simulink model "atrias_system_testing_delay"  (R2014a)
settings: Solver=FixedStepDiscrete  StartTime=0.0  StopTime=inf  FixedStep=sample_time  RelTol=1e-3
PreLoadFcn:
  | set_sampletime
PostLoadFcn:
  | set_sampletime
InitFcn:
  | sys_params
StartFcn:
  | set_sampletime
values from neighbouring files (symbols this model uses):
  A_lpf_velocity = 1 + B1_lpf_velocity + B2_lpf_velocity    [daq_params_osu.m]
  B1_lpf_velocity = -2*exp(-lpf_damping*fcut_velocity*sample_time)*cos(fcut_velocity*sample_time*sqrt(1-lpf_damping^2))    [daq_params_osu.m]
  B2_lpf_velocity = exp(-2*lpf_damping*fcut_velocity*sample_time)    [daq_params_osu.m]
  BOOM_MAX_ENCODER_TICKS = 2^17 - 1    (= 131071)    [daq_params_osu.m]
  BOOM_PITCH_CAL_VALUE_RAD = 0    [daq_params_osu.m]
  BOOM_PITCH_CAL_VALUE_TICKS = 43809    [daq_params_osu.m]
  BOOM_PITCH_ENCODER_RAD_PER_TICK = -2*pi / (2^17 * 2)    (= -2.39684498107e-05)    [daq_params_osu.m]
  BOOM_ROLL_CAL_VALUE_RAD = 0.1271    [daq_params_osu.m]
  BOOM_ROLL_CAL_VALUE_TICKS = 9318    [daq_params_osu.m]
  BOOM_ROLL_ENCODER_RAD_PER_TICK = 2*pi / (2^17 * 7)    (= 6.84812851735e-06)    [daq_params_osu.m]
  BOOM_YAW_ENCODER_RAD_PER_TICK = 2*pi / (2^17 * 9.6)    (= 4.9934270439e-06)    [daq_params_osu.m]
  CURRENT_LIMIT = 100    [daq_params_osu.m]
  fcut_smooth = 16*(2*pi)    (= 100.530964915)    [daq_params_osu.m]
  fcut_unwrap = 8*(2*pi)    (= 50.2654824574)    [daq_params_osu.m]
  gui_disable_cmd = 0    [daq_params_osu.m]
  gui_enable_cmd = 0    [daq_params_osu.m]
  gui_estop_cmd = 0    [daq_params_osu.m]
  gui_reset_cmd = 0    [daq_params_osu.m]
  HIP_ABS_ENCODER_RAD_PER_TICK = 2*pi / 2^13    (= 0.000766990393943)    [daq_params_osu.m]
  HIP_ABS_MAX_ENCODER_TICKS = 2^13 - 1    (= 8191)    [daq_params_osu.m]
  HIP_INC_ENCODER_RAD_PER_TICK = 2*pi / (2500 * 4 * 57)    (= 1.10231321179e-05)    [daq_params_osu.m]
  HIP_INC_MAX_ENCODER_TICKS = 2^16 - 1    (= 65535)    [daq_params_osu.m]
  HIP_MOTOR_CONSTANT = 0.184    [daq_params_osu.m]
  HIP_MTR_GEAR_RATIO = 57    [daq_params_osu.m]
  HIP_MTR_MAX_TORQUE = MTR_HIP_MAX_CURRENT*HIP_MOTOR_CONSTANT*HIP_MTR_GEAR_RATIO    (= 629.28)    [daq_params_osu.m]
  INC_ENC_DIRS = -[ LEG1_MOTOR_A_DIRECTION ... (first row only)    [daq_params_osu.m]
  INC_ENC_RAD_PER_TICK = 2*pi/14000/LEG_MTR_GEAR_RATIO    (= 8.97597901026e-06)    [daq_params_osu.m]
  k_sea = 4118    [sys_params.m]
  LEFT_HIP_CALIB_POS = 0    [daq_params_osu.m]
  LEFT_HIP_CALIB_VAL = 7192 - 2^13    (= -1000)    [daq_params_osu.m]
  LEFT_MOTOR_HIP_DIRECTION = -1.0    (= -1)    [daq_params_osu.m]
  LEG1_LEG_A_CALIB_VAL = 265417675    [daq_params_osu.m]
  LEG1_LEG_A_RAD_PER_CNT = -9.8039216e-09    [daq_params_osu.m]
  LEG1_LEG_B_CALIB_VAL = 175319150    [daq_params_osu.m]
  LEG1_LEG_B_RAD_PER_CNT = -9.8039216e-09    [daq_params_osu.m]
  LEG1_MOTOR_A_DIRECTION = -1.0    (= -1)    [daq_params_osu.m]
  LEG1_MOTOR_B_DIRECTION = -1.0    (= -1)    [daq_params_osu.m]
  LEG1_TRAN_A_CALIB_VAL = 143046540    [daq_params_osu.m]
  LEG1_TRAN_A_RAD_PER_CNT = 9.8039216e-09    [daq_params_osu.m]
  LEG1_TRAN_B_CALIB_VAL = 142356572    [daq_params_osu.m]
  LEG1_TRAN_B_RAD_PER_CNT = -9.8039216e-09    [daq_params_osu.m]
  LEG2_LEG_A_CALIB_VAL = 264357825    [daq_params_osu.m]
  LEG2_LEG_A_RAD_PER_CNT = -9.8039216e-09    [daq_params_osu.m]
  LEG2_LEG_B_CALIB_VAL = 261444054    [daq_params_osu.m]
  LEG2_LEG_B_RAD_PER_CNT = 9.8039216e-09    [daq_params_osu.m]
  LEG2_MOTOR_A_DIRECTION = 1.0    (= 1)    [daq_params_osu.m]
  LEG2_MOTOR_B_DIRECTION = 1.0    (= 1)    [daq_params_osu.m]
  LEG2_TRAN_A_CALIB_VAL = 142300933    [daq_params_osu.m]
  LEG2_TRAN_A_RAD_PER_CNT = 9.8039216e-09    [daq_params_osu.m]
  LEG2_TRAN_B_CALIB_VAL = 142287413    [daq_params_osu.m]
  LEG2_TRAN_B_RAD_PER_CNT = -9.8039216e-09    [daq_params_osu.m]
  LEG_A_CALIB_LOC = pi + 0.305432619099008    (= 3.44702527269)    [daq_params_osu.m]
  LEG_B_CALIB_LOC = pi - 0.305432619099008    (= 2.83616003449)    [daq_params_osu.m]
  LEG_MOTOR_CONSTANT = 0.119    [daq_params_osu.m]
  LEG_MTR_GEAR_RATIO = 50    [daq_params_osu.m]
  LEG_MTR_MAX_TORQUE = MTR_MAX_CURRENT*LEG_MOTOR_CONSTANT*LEG_MTR_GEAR_RATIO    (= 922.25)    [daq_params_osu.m]
  max_encoder_velocity = 200    [daq_params_osu.m]
  MEDULLA_ADC_MAX_VOLTS = 2.70    (= 2.7)    [daq_params_osu.m]
  MEDULLA_ADC_OFFSET_COUNTS = 172    [daq_params_osu.m]
  MEDULLA_STATE_ERROR = 5    [daq_params_osu.m]
  MEDULLA_STATE_HALT = 4    [daq_params_osu.m]
  MEDULLA_STATE_IDLE = 0    [daq_params_osu.m]
  MEDULLA_STATE_RESET = 6    [daq_params_osu.m]
  MEDULLA_STATE_RUN = 2    [daq_params_osu.m]
  MEDULLA_TIMER_FREQ = 32e6    (= 32000000)    [daq_params_osu.m]
  MOTOR_POSITION_LIMITS_LOWER = [2.5; 1.4; 0.4]    [daq_params_osu.m]
  MOTOR_POSITION_LIMITS_UPPER = [4.9; 3.8; 2.5]    [daq_params_osu.m]
  MTR_HIP_MAX_CURRENT = 60.0    (= 60)    [daq_params_osu.m]
  MTR_MAX_CONT_CURRENT = 100.0    (= 100)    [daq_params_osu.m]
  MTR_MAX_COUNT = 19900    [daq_params_osu.m]
  MTR_MAX_CURRENT = 155.0    (= 155)    [daq_params_osu.m]
  nom_sample_time = 0.001    [sys_params.m]
  RIGHT_HIP_CALIB_POS = 0    [daq_params_osu.m]
  RIGHT_HIP_CALIB_VAL = 1091    [daq_params_osu.m]
  RIGHT_MOTOR_HIP_DIRECTION = 1.0    (= 1)    [daq_params_osu.m]
  sample_time = 1/update_freq    (= 0.001)    [daq_params_osu.m]
  sensor_start_time = 8    [daq_params_osu.m]
undefined symbols (not defined in the file or in its folder): max_sensor_velocity
libraries: xpcethercatlib x196, simulink x50, slrtlib x4, dspswit3 x1
(part 3 of 4)

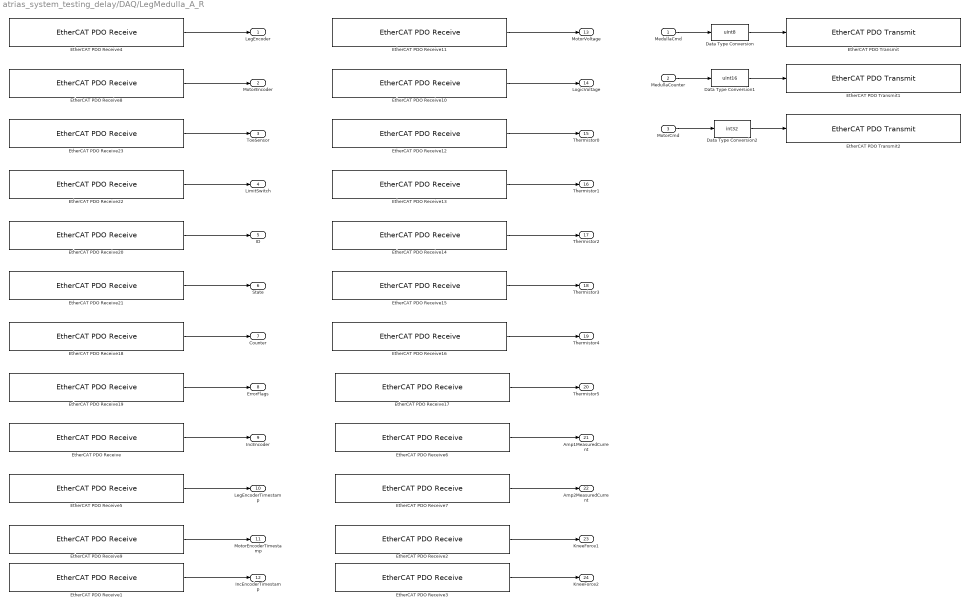
== system atrias_system_testing_delay/DAQ/LegMedulla_A_R ==
  MedullaCmd : Inport
  MedullaCounter : Inport  Port=2
  MotorCmd : Inport  Port=3
  Data Type Conversion : DataTypeConversion  OutDataTypeStr=uint8
  Data Type Conversion1 : DataTypeConversion  OutDataTypeStr=uint16
  Data Type Conversion2 : DataTypeConversion  OutDataTypeStr=int32
  EtherCAT PDO Receive : xpcethercatlib/EtherCAT PDO Receive  Priority=2  sig_name=Box 7 (ATRIAS 2.1 Leg (Medulla 1.5)).Incremental Encoder.Incremental Encoder  sig_offset=2120  sig_type=uint16  type_size=16  sig_dim=1  device_id=0  sample_time=0.001000
  EtherCAT PDO Receive1 : xpcethercatlib/EtherCAT PDO Receive  Priority=2  sig_name=Box 7 (ATRIAS 2.1 Leg (Medulla 1.5)).Incremental Encoder.Incremental Encoder Timestamp  sig_offset=2136  sig_type=uint16  type_size=16  sig_dim=1  device_id=0  sample_time=0.001000
  EtherCAT PDO Receive10 : xpcethercatlib/EtherCAT PDO Receive  Priority=2  sig_name=Box 7 (ATRIAS 2.1 Leg (Medulla 1.5)).Power.Logic Voltage  sig_offset=2168  sig_type=uint16  type_size=16  sig_dim=1  device_id=0  sample_time=0.001000
  EtherCAT PDO Receive11 : xpcethercatlib/EtherCAT PDO Receive  Priority=2  sig_name=Box 7 (ATRIAS 2.1 Leg (Medulla 1.5)).Power.Motor Voltage  sig_offset=2152  sig_type=uint16  type_size=16  sig_dim=1  device_id=0  sample_time=0.001000
  EtherCAT PDO Receive12 : xpcethercatlib/EtherCAT PDO Receive  Priority=2  sig_name=Box 7 (ATRIAS 2.1 Leg (Medulla 1.5)).Thermistors.Thermistor 0  sig_offset=2184  sig_type=uint16  type_size=16  sig_dim=1  device_id=0  sample_time=0.001000
  EtherCAT PDO Receive13 : xpcethercatlib/EtherCAT PDO Receive  Priority=2  sig_name=Box 7 (ATRIAS 2.1 Leg (Medulla 1.5)).Thermistors.Thermistor 1  sig_offset=2200  sig_type=uint16  type_size=16  sig_dim=1  device_id=0  sample_time=0.001000
  EtherCAT PDO Receive14 : xpcethercatlib/EtherCAT PDO Receive  Priority=2  sig_name=Box 7 (ATRIAS 2.1 Leg (Medulla 1.5)).Thermistors.Thermistor 2  sig_offset=2216  sig_type=uint16  type_size=16  sig_dim=1  device_id=0  sample_time=0.001000
  EtherCAT PDO Receive15 : xpcethercatlib/EtherCAT PDO Receive  Priority=2  sig_name=Box 7 (ATRIAS 2.1 Leg (Medulla 1.5)).Thermistors.Thermistor 3  sig_offset=2232  sig_type=uint16  type_size=16  sig_dim=1  device_id=0  sample_time=0.001000
  EtherCAT PDO Receive16 : xpcethercatlib/EtherCAT PDO Receive  Priority=2  sig_name=Box 7 (ATRIAS 2.1 Leg (Medulla 1.5)).Thermistors.Thermistor 4  sig_offset=2248  sig_type=uint16  type_size=16  sig_dim=1  device_id=0  sample_time=0.001000
  EtherCAT PDO Receive17 : xpcethercatlib/EtherCAT PDO Receive  Priority=2  sig_name=Box 7 (ATRIAS 2.1 Leg (Medulla 1.5)).Thermistors.Thermistor 5  sig_offset=2264  sig_type=uint16  type_size=16  sig_dim=1  device_id=0  sample_time=0.001000
  EtherCAT PDO Receive18 : xpcethercatlib/EtherCAT PDO Receive  Priority=2  sig_name=Box 7 (ATRIAS 2.1 Leg (Medulla 1.5)).uController Status.Counter  sig_offset=1984  sig_type=uint8  type_size=8  sig_dim=1  device_id=0  sample_time=0.001000
  EtherCAT PDO Receive19 : xpcethercatlib/EtherCAT PDO Receive  Priority=2  sig_name=Box 7 (ATRIAS 2.1 Leg (Medulla 1.5)).uController Status.Error Flags  sig_offset=1992  sig_type=uint8  type_size=8  sig_dim=1  device_id=0  sample_time=0.001000
  EtherCAT PDO Receive2 : xpcethercatlib/EtherCAT PDO Receive  Priority=2  sig_name=Box 7 (ATRIAS 2.1 Leg (Medulla 1.5)).Knee Force.Knee Force 1  sig_offset=2312  sig_type=uint16  type_size=16  sig_dim=1  device_id=0  sample_time=0.001000
  EtherCAT PDO Receive20 : xpcethercatlib/EtherCAT PDO Receive  Priority=2  sig_name=Box 7 (ATRIAS 2.1 Leg (Medulla 1.5)).uController Status.ID  sig_offset=1968  sig_type=uint8  type_size=8  sig_dim=1  device_id=0  sample_time=0.001000
  EtherCAT PDO Receive21 : xpcethercatlib/EtherCAT PDO Receive  Priority=2  sig_name=Box 7 (ATRIAS 2.1 Leg (Medulla 1.5)).uController Status.State  sig_offset=1976  sig_type=uint8  type_size=8  sig_dim=1  device_id=0  sample_time=0.001000
  EtherCAT PDO Receive22 : xpcethercatlib/EtherCAT PDO Receive  Priority=2  sig_name=Box 7 (ATRIAS 2.1 Leg (Medulla 1.5)).uController Status.Limit Switch  sig_offset=2000  sig_type=uint8  type_size=8  sig_dim=1  device_id=0  sample_time=0.001000
  EtherCAT PDO Receive23 : xpcethercatlib/EtherCAT PDO Receive  Priority=2  sig_name=Box 7 (ATRIAS 2.1 Leg (Medulla 1.5)).uController Status.Toe Sensor  sig_offset=2008  sig_type=uint16  type_size=16  sig_dim=1  device_id=0  sample_time=0.001000
  EtherCAT PDO Receive3 : xpcethercatlib/EtherCAT PDO Receive  Priority=2  sig_name=Box 7 (ATRIAS 2.1 Leg (Medulla 1.5)).Knee Force.Knee Force 2  sig_offset=2328  sig_type=uint16  type_size=16  sig_dim=1  device_id=0  sample_time=0.001000
  EtherCAT PDO Receive4 : xpcethercatlib/EtherCAT PDO Receive  Priority=2  sig_name=Box 7 (ATRIAS 2.1 Leg (Medulla 1.5)).Leg Encoder.Leg Encoder  sig_offset=2072  sig_type=uint32  type_size=32  sig_dim=1  device_id=0  sample_time=0.001000
  EtherCAT PDO Receive5 : xpcethercatlib/EtherCAT PDO Receive  Priority=2  sig_name=Box 7 (ATRIAS 2.1 Leg (Medulla 1.5)).Leg Encoder.Leg Encoder Timestamp  sig_offset=2104  sig_type=uint16  type_size=16  sig_dim=1  device_id=0  sample_time=0.001000
  EtherCAT PDO Receive6 : xpcethercatlib/EtherCAT PDO Receive  Priority=2  sig_name=Box 7 (ATRIAS 2.1 Leg (Medulla 1.5)).Measured Current.Amp 1 Measured Current  sig_offset=2280  sig_type=int16  type_size=16  sig_dim=1  device_id=0  sample_time=0.001000
  EtherCAT PDO Receive7 : xpcethercatlib/EtherCAT PDO Receive  Priority=2  sig_name=Box 7 (ATRIAS 2.1 Leg (Medulla 1.5)).Measured Current.Amp 2 Measured Current  sig_offset=2296  sig_type=int16  type_size=16  sig_dim=1  device_id=0  sample_time=0.001000
  EtherCAT PDO Receive8 : xpcethercatlib/EtherCAT PDO Receive  Priority=2  sig_name=Box 7 (ATRIAS 2.1 Leg (Medulla 1.5)).Motor Encoder.Motor Encoder  sig_offset=2024  sig_type=uint32  type_size=32  sig_dim=1  device_id=0  sample_time=0.001000
  EtherCAT PDO Receive9 : xpcethercatlib/EtherCAT PDO Receive  Priority=2  sig_name=Box 7 (ATRIAS 2.1 Leg (Medulla 1.5)).Motor Encoder.Motor Encoder Timestamp  sig_offset=2056  sig_type=uint16  type_size=16  sig_dim=1  device_id=0  sample_time=0.001000
  EtherCAT PDO Transmit : xpcethercatlib/EtherCAT PDO Transmit   Priority=3  sig_name=Box 7 (ATRIAS 2.1 Leg (Medulla 1.5)).uControllerInput.Command  sig_offset=1968  sig_type=uint8  type_size=8  sig_dim=1  device_id=0  sample_time=0.001000
  EtherCAT PDO Transmit1 : xpcethercatlib/EtherCAT PDO Transmit   Priority=3  sig_name=Box 7 (ATRIAS 2.1 Leg (Medulla 1.5)).uControllerInput.Counter  sig_offset=1976  sig_type=uint16  type_size=16  sig_dim=1  device_id=0  sample_time=0.001000
  EtherCAT PDO Transmit2 : xpcethercatlib/EtherCAT PDO Transmit   Priority=3  sig_name=Box 7 (ATRIAS 2.1 Leg (Medulla 1.5)).uControllerInput.Motor Current  sig_offset=1992  sig_type=int32  type_size=32  sig_dim=1  device_id=0  sample_time=0.001000
  LegEncoder : Outport
  MotorEncoder : Outport  Port=2
  ToeSensor : Outport  Port=3
  LimitSwitch : Outport  Port=4
  ID : Outport  Port=5
  State : Outport  Port=6
  Counter : Outport  Port=7
  ErrorFlags : Outport  Port=8
  IncEncoder : Outport  Port=9
  LegEncoderTimestamp : Outport  Port=10
  MotorEncoderTimestamp : Outport  Port=11
  IncEncoderTimestamp : Outport  Port=12
  MotorVoltage : Outport  Port=13
  LogicVoltage : Outport  Port=14
  Thermistor0 : Outport  Port=15
  Thermistor1 : Outport  Port=16
  Thermistor2 : Outport  Port=17
  Thermistor3 : Outport  Port=18
  Thermistor4 : Outport  Port=19
  Thermistor5 : Outport  Port=20
  Amp1MeasuredCurrent : Outport  Port=21
  Amp2MeasuredCurrent : Outport  Port=22
  KneeForce1 : Outport  Port=23
  KneeForce2 : Outport  Port=24
  wires:
  Data Type Conversion/1 -> EtherCAT PDO Transmit/1
  Data Type Conversion1/1 -> EtherCAT PDO Transmit1/1
  Data Type Conversion2/1 -> EtherCAT PDO Transmit2/1
  EtherCAT PDO Receive/1 -> IncEncoder/1
  EtherCAT PDO Receive1/1 -> IncEncoderTimestamp/1
  EtherCAT PDO Receive2/1 -> KneeForce1/1
  EtherCAT PDO Receive3/1 -> KneeForce2/1
  EtherCAT PDO Receive4/1 -> LegEncoder/1
  EtherCAT PDO Receive5/1 -> LegEncoderTimestamp/1
  EtherCAT PDO Receive6/1 -> Amp1MeasuredCurrent/1
  EtherCAT PDO Receive7/1 -> Amp2MeasuredCurrent/1
  EtherCAT PDO Receive8/1 -> MotorEncoder/1
  EtherCAT PDO Receive9/1 -> MotorEncoderTimestamp/1
  EtherCAT PDO Receive10/1 -> LogicVoltage/1
  EtherCAT PDO Receive11/1 -> MotorVoltage/1
  EtherCAT PDO Receive12/1 -> Thermistor0/1
  EtherCAT PDO Receive13/1 -> Thermistor1/1
  EtherCAT PDO Receive14/1 -> Thermistor2/1
  EtherCAT PDO Receive15/1 -> Thermistor3/1
  EtherCAT PDO Receive16/1 -> Thermistor4/1
  EtherCAT PDO Receive17/1 -> Thermistor5/1
  EtherCAT PDO Receive18/1 -> Counter/1
  EtherCAT PDO Receive19/1 -> ErrorFlags/1
  EtherCAT PDO Receive20/1 -> ID/1
  EtherCAT PDO Receive22/1 -> LimitSwitch/1
  EtherCAT PDO Receive21/1 -> State/1
  EtherCAT PDO Receive23/1 -> ToeSensor/1
  MedullaCmd/1 -> Data Type Conversion/1
  MedullaCounter/1 -> Data Type Conversion1/1
  MotorCmd/1 -> Data Type Conversion2/1

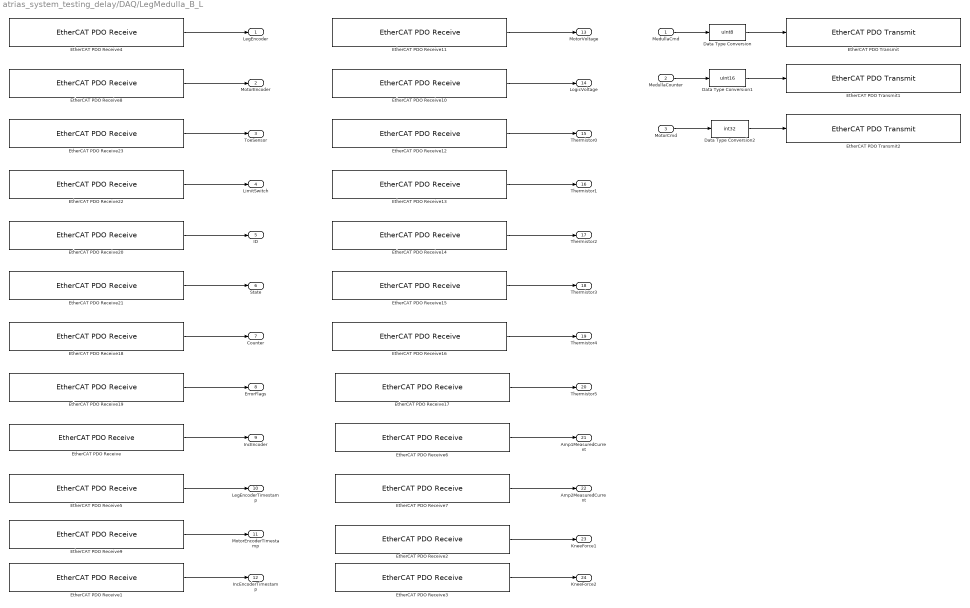
== system atrias_system_testing_delay/DAQ/LegMedulla_B_L ==
  MedullaCmd : Inport
  MedullaCounter : Inport  Port=2
  MotorCmd : Inport  Port=3
  Data Type Conversion : DataTypeConversion  OutDataTypeStr=uint8
  Data Type Conversion1 : DataTypeConversion  OutDataTypeStr=uint16
  Data Type Conversion2 : DataTypeConversion  OutDataTypeStr=int32
  EtherCAT PDO Receive : xpcethercatlib/EtherCAT PDO Receive  Priority=2  sig_name=Box 5 (ATRIAS 2.1 Leg (Medulla 1.5)).Incremental Encoder.Incremental Encoder  sig_offset=1368  sig_type=uint16  type_size=16  sig_dim=1  device_id=0  sample_time=0.001000
  EtherCAT PDO Receive1 : xpcethercatlib/EtherCAT PDO Receive  Priority=2  sig_name=Box 5 (ATRIAS 2.1 Leg (Medulla 1.5)).Incremental Encoder.Incremental Encoder Timestamp  sig_offset=1384  sig_type=uint16  type_size=16  sig_dim=1  device_id=0  sample_time=0.001000
  EtherCAT PDO Receive10 : xpcethercatlib/EtherCAT PDO Receive  Priority=2  sig_name=Box 5 (ATRIAS 2.1 Leg (Medulla 1.5)).Power.Logic Voltage  sig_offset=1416  sig_type=uint16  type_size=16  sig_dim=1  device_id=0  sample_time=0.001000
  EtherCAT PDO Receive11 : xpcethercatlib/EtherCAT PDO Receive  Priority=2  sig_name=Box 5 (ATRIAS 2.1 Leg (Medulla 1.5)).Power.Motor Voltage  sig_offset=1400  sig_type=uint16  type_size=16  sig_dim=1  device_id=0  sample_time=0.001000
  EtherCAT PDO Receive12 : xpcethercatlib/EtherCAT PDO Receive  Priority=2  sig_name=Box 5 (ATRIAS 2.1 Leg (Medulla 1.5)).Thermistors.Thermistor 0  sig_offset=1432  sig_type=uint16  type_size=16  sig_dim=1  device_id=0  sample_time=0.001000
  EtherCAT PDO Receive13 : xpcethercatlib/EtherCAT PDO Receive  Priority=2  sig_name=Box 5 (ATRIAS 2.1 Leg (Medulla 1.5)).Thermistors.Thermistor 1  sig_offset=1448  sig_type=uint16  type_size=16  sig_dim=1  device_id=0  sample_time=0.001000
  EtherCAT PDO Receive14 : xpcethercatlib/EtherCAT PDO Receive  Priority=2  sig_name=Box 5 (ATRIAS 2.1 Leg (Medulla 1.5)).Thermistors.Thermistor 2  sig_offset=1464  sig_type=uint16  type_size=16  sig_dim=1  device_id=0  sample_time=0.001000
  EtherCAT PDO Receive15 : xpcethercatlib/EtherCAT PDO Receive  Priority=2  sig_name=Box 5 (ATRIAS 2.1 Leg (Medulla 1.5)).Thermistors.Thermistor 3  sig_offset=1480  sig_type=uint16  type_size=16  sig_dim=1  device_id=0  sample_time=0.001000
  EtherCAT PDO Receive16 : xpcethercatlib/EtherCAT PDO Receive  Priority=2  sig_name=Box 5 (ATRIAS 2.1 Leg (Medulla 1.5)).Thermistors.Thermistor 4  sig_offset=1496  sig_type=uint16  type_size=16  sig_dim=1  device_id=0  sample_time=0.001000
  EtherCAT PDO Receive17 : xpcethercatlib/EtherCAT PDO Receive  Priority=2  sig_name=Box 5 (ATRIAS 2.1 Leg (Medulla 1.5)).Thermistors.Thermistor 5  sig_offset=1512  sig_type=uint16  type_size=16  sig_dim=1  device_id=0  sample_time=0.001000
  EtherCAT PDO Receive18 : xpcethercatlib/EtherCAT PDO Receive  Priority=2  sig_name=Box 5 (ATRIAS 2.1 Leg (Medulla 1.5)).uController Status.Counter  sig_offset=1232  sig_type=uint8  type_size=8  sig_dim=1  device_id=0  sample_time=0.001000
  EtherCAT PDO Receive19 : xpcethercatlib/EtherCAT PDO Receive  Priority=2  sig_name=Box 5 (ATRIAS 2.1 Leg (Medulla 1.5)).uController Status.Error Flags  sig_offset=1240  sig_type=uint8  type_size=8  sig_dim=1  device_id=0  sample_time=0.001000
  EtherCAT PDO Receive2 : xpcethercatlib/EtherCAT PDO Receive  Priority=2  sig_name=Box 5 (ATRIAS 2.1 Leg (Medulla 1.5)).Knee Force.Knee Force 1  sig_offset=1560  sig_type=uint16  type_size=16  sig_dim=1  device_id=0  sample_time=0.001000
  EtherCAT PDO Receive20 : xpcethercatlib/EtherCAT PDO Receive  Priority=2  sig_name=Box 5 (ATRIAS 2.1 Leg (Medulla 1.5)).uController Status.ID  sig_offset=1216  sig_type=uint8  type_size=8  sig_dim=1  device_id=0  sample_time=0.001000
  EtherCAT PDO Receive21 : xpcethercatlib/EtherCAT PDO Receive  Priority=2  sig_name=Box 5 (ATRIAS 2.1 Leg (Medulla 1.5)).uController Status.State  sig_offset=1224  sig_type=uint8  type_size=8  sig_dim=1  device_id=0  sample_time=0.001000
  EtherCAT PDO Receive22 : xpcethercatlib/EtherCAT PDO Receive  Priority=2  sig_name=Box 5 (ATRIAS 2.1 Leg (Medulla 1.5)).uController Status.Limit Switch  sig_offset=1248  sig_type=uint8  type_size=8  sig_dim=1  device_id=0  sample_time=0.001000
  EtherCAT PDO Receive23 : xpcethercatlib/EtherCAT PDO Receive  Priority=2  sig_name=Box 5 (ATRIAS 2.1 Leg (Medulla 1.5)).uController Status.Toe Sensor  sig_offset=1256  sig_type=uint16  type_size=16  sig_dim=1  device_id=0  sample_time=0.001000
  EtherCAT PDO Receive3 : xpcethercatlib/EtherCAT PDO Receive  Priority=2  sig_name=Box 5 (ATRIAS 2.1 Leg (Medulla 1.5)).Knee Force.Knee Force 2  sig_offset=1576  sig_type=uint16  type_size=16  sig_dim=1  device_id=0  sample_time=0.001000
  EtherCAT PDO Receive4 : xpcethercatlib/EtherCAT PDO Receive  Priority=2  sig_name=Box 5 (ATRIAS 2.1 Leg (Medulla 1.5)).Leg Encoder.Leg Encoder  sig_offset=1320  sig_type=uint32  type_size=32  sig_dim=1  device_id=0  sample_time=0.001000
  EtherCAT PDO Receive5 : xpcethercatlib/EtherCAT PDO Receive  Priority=2  sig_name=Box 5 (ATRIAS 2.1 Leg (Medulla 1.5)).Leg Encoder.Leg Encoder Timestamp  sig_offset=1352  sig_type=uint16  type_size=16  sig_dim=1  device_id=0  sample_time=0.001000
  EtherCAT PDO Receive6 : xpcethercatlib/EtherCAT PDO Receive  Priority=2  sig_name=Box 5 (ATRIAS 2.1 Leg (Medulla 1.5)).Measured Current.Amp 1 Measured Current  sig_offset=1528  sig_type=int16  type_size=16  sig_dim=1  device_id=0  sample_time=0.001000
  EtherCAT PDO Receive7 : xpcethercatlib/EtherCAT PDO Receive  Priority=2  sig_name=Box 5 (ATRIAS 2.1 Leg (Medulla 1.5)).Measured Current.Amp 2 Measured Current  sig_offset=1544  sig_type=int16  type_size=16  sig_dim=1  device_id=0  sample_time=0.001000
  EtherCAT PDO Receive8 : xpcethercatlib/EtherCAT PDO Receive  Priority=2  sig_name=Box 5 (ATRIAS 2.1 Leg (Medulla 1.5)).Motor Encoder.Motor Encoder  sig_offset=1272  sig_type=uint32  type_size=32  sig_dim=1  device_id=0  sample_time=0.001000
  EtherCAT PDO Receive9 : xpcethercatlib/EtherCAT PDO Receive  Priority=2  sig_name=Box 5 (ATRIAS 2.1 Leg (Medulla 1.5)).Motor Encoder.Motor Encoder Timestamp  sig_offset=1304  sig_type=uint16  type_size=16  sig_dim=1  device_id=0  sample_time=0.001000
  EtherCAT PDO Transmit : xpcethercatlib/EtherCAT PDO Transmit   Priority=3  sig_name=Box 5 (ATRIAS 2.1 Leg (Medulla 1.5)).uControllerInput.Command  sig_offset=1216  sig_type=uint8  type_size=8  sig_dim=1  device_id=0  sample_time=0.001000
  EtherCAT PDO Transmit1 : xpcethercatlib/EtherCAT PDO Transmit   Priority=3  sig_name=Box 5 (ATRIAS 2.1 Leg (Medulla 1.5)).uControllerInput.Counter  sig_offset=1224  sig_type=uint16  type_size=16  sig_dim=1  device_id=0  sample_time=0.001000
  EtherCAT PDO Transmit2 : xpcethercatlib/EtherCAT PDO Transmit   Priority=3  sig_name=Box 5 (ATRIAS 2.1 Leg (Medulla 1.5)).uControllerInput.Motor Current  sig_offset=1240  sig_type=int32  type_size=32  sig_dim=1  device_id=0  sample_time=0.001000
  LegEncoder : Outport
  MotorEncoder : Outport  Port=2
  ToeSensor : Outport  Port=3
  LimitSwitch : Outport  Port=4
  ID : Outport  Port=5
  State : Outport  Port=6
  Counter : Outport  Port=7
  ErrorFlags : Outport  Port=8
  IncEncoder : Outport  Port=9
  LegEncoderTimestamp : Outport  Port=10
  MotorEncoderTimestamp : Outport  Port=11
  IncEncoderTimestamp : Outport  Port=12
  MotorVoltage : Outport  Port=13
  LogicVoltage : Outport  Port=14
  Thermistor0 : Outport  Port=15
  Thermistor1 : Outport  Port=16
  Thermistor2 : Outport  Port=17
  Thermistor3 : Outport  Port=18
  Thermistor4 : Outport  Port=19
  Thermistor5 : Outport  Port=20
  Amp1MeasuredCurrent : Outport  Port=21
  Amp2MeasuredCurrent : Outport  Port=22
  KneeForce1 : Outport  Port=23
  KneeForce2 : Outport  Port=24
  wires:
  Data Type Conversion/1 -> EtherCAT PDO Transmit/1
  Data Type Conversion1/1 -> EtherCAT PDO Transmit1/1
  Data Type Conversion2/1 -> EtherCAT PDO Transmit2/1
  EtherCAT PDO Receive/1 -> IncEncoder/1
  EtherCAT PDO Receive1/1 -> IncEncoderTimestamp/1
  EtherCAT PDO Receive2/1 -> KneeForce1/1
  EtherCAT PDO Receive3/1 -> KneeForce2/1
  EtherCAT PDO Receive4/1 -> LegEncoder/1
  EtherCAT PDO Receive5/1 -> LegEncoderTimestamp/1
  EtherCAT PDO Receive6/1 -> Amp1MeasuredCurrent/1
  EtherCAT PDO Receive7/1 -> Amp2MeasuredCurrent/1
  EtherCAT PDO Receive8/1 -> MotorEncoder/1
  EtherCAT PDO Receive9/1 -> MotorEncoderTimestamp/1
  EtherCAT PDO Receive10/1 -> LogicVoltage/1
  EtherCAT PDO Receive11/1 -> MotorVoltage/1
  EtherCAT PDO Receive12/1 -> Thermistor0/1
  EtherCAT PDO Receive13/1 -> Thermistor1/1
  EtherCAT PDO Receive14/1 -> Thermistor2/1
  EtherCAT PDO Receive15/1 -> Thermistor3/1
  EtherCAT PDO Receive16/1 -> Thermistor4/1
  EtherCAT PDO Receive17/1 -> Thermistor5/1
  EtherCAT PDO Receive18/1 -> Counter/1
  EtherCAT PDO Receive19/1 -> ErrorFlags/1
  EtherCAT PDO Receive20/1 -> ID/1
  EtherCAT PDO Receive22/1 -> LimitSwitch/1
  EtherCAT PDO Receive21/1 -> State/1
  EtherCAT PDO Receive23/1 -> ToeSensor/1
  MedullaCmd/1 -> Data Type Conversion/1
  MedullaCounter/1 -> Data Type Conversion1/1
  MotorCmd/1 -> Data Type Conversion2/1

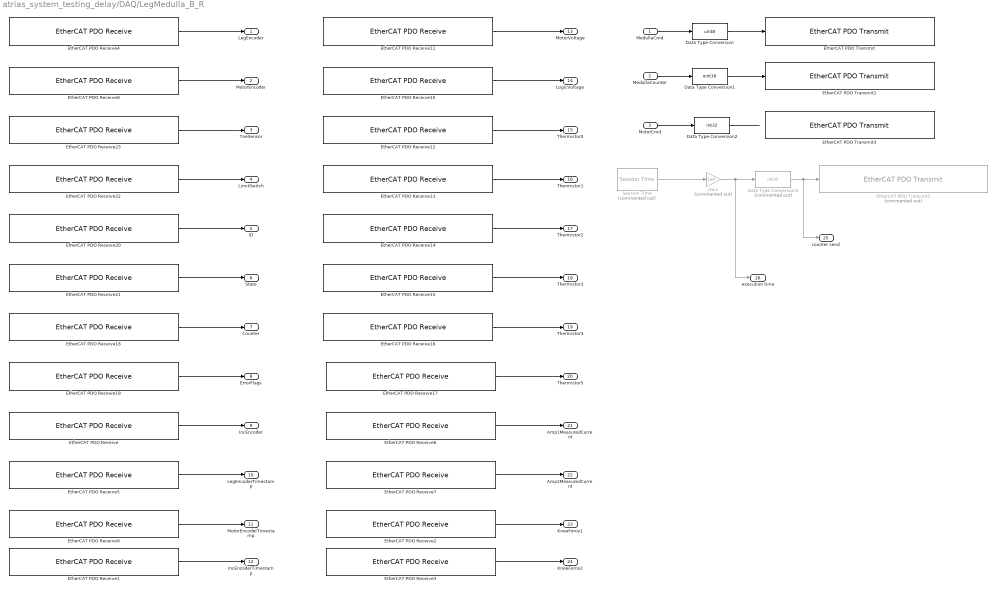
== system atrias_system_testing_delay/DAQ/LegMedulla_B_R ==
  MedullaCmd : Inport
  MedullaCounter : Inport  Port=2
  MotorCmd : Inport  Port=3
  Data Type Conversion : DataTypeConversion  OutDataTypeStr=uint8
  Data Type Conversion1 : DataTypeConversion  OutDataTypeStr=uint16
  Data Type Conversion2 : DataTypeConversion  OutDataTypeStr=int32
  Data Type Conversion3 : DataTypeConversion  Commented=on  OutDataTypeStr=int32
  EtherCAT PDO Receive : xpcethercatlib/EtherCAT PDO Receive  Priority=2  sig_name=Box 6 (ATRIAS 2.1 Leg (Medulla 1.5)).Incremental Encoder.Incremental Encoder  sig_offset=1744  sig_type=uint16  type_size=16  sig_dim=1  device_id=0  sample_time=0.001000
  EtherCAT PDO Receive1 : xpcethercatlib/EtherCAT PDO Receive  Priority=2  sig_name=Box 6 (ATRIAS 2.1 Leg (Medulla 1.5)).Incremental Encoder.Incremental Encoder Timestamp  sig_offset=1760  sig_type=uint16  type_size=16  sig_dim=1  device_id=0  sample_time=0.001000
  EtherCAT PDO Receive10 : xpcethercatlib/EtherCAT PDO Receive  Priority=2  sig_name=Box 6 (ATRIAS 2.1 Leg (Medulla 1.5)).Power.Logic Voltage  sig_offset=1792  sig_type=uint16  type_size=16  sig_dim=1  device_id=0  sample_time=0.001000
  EtherCAT PDO Receive11 : xpcethercatlib/EtherCAT PDO Receive  Priority=2  sig_name=Box 6 (ATRIAS 2.1 Leg (Medulla 1.5)).Power.Motor Voltage  sig_offset=1776  sig_type=uint16  type_size=16  sig_dim=1  device_id=0  sample_time=0.001000
  EtherCAT PDO Receive12 : xpcethercatlib/EtherCAT PDO Receive  Priority=2  sig_name=Box 6 (ATRIAS 2.1 Leg (Medulla 1.5)).Thermistors.Thermistor 0  sig_offset=1808  sig_type=uint16  type_size=16  sig_dim=1  device_id=0  sample_time=0.001000
  EtherCAT PDO Receive13 : xpcethercatlib/EtherCAT PDO Receive  Priority=2  sig_name=Box 6 (ATRIAS 2.1 Leg (Medulla 1.5)).Thermistors.Thermistor 1  sig_offset=1824  sig_type=uint16  type_size=16  sig_dim=1  device_id=0  sample_time=0.001000
  EtherCAT PDO Receive14 : xpcethercatlib/EtherCAT PDO Receive  Priority=2  sig_name=Box 6 (ATRIAS 2.1 Leg (Medulla 1.5)).Thermistors.Thermistor 2  sig_offset=1840  sig_type=uint16  type_size=16  sig_dim=1  device_id=0  sample_time=0.001000
  EtherCAT PDO Receive15 : xpcethercatlib/EtherCAT PDO Receive  Priority=2  sig_name=Box 6 (ATRIAS 2.1 Leg (Medulla 1.5)).Thermistors.Thermistor 3  sig_offset=1856  sig_type=uint16  type_size=16  sig_dim=1  device_id=0  sample_time=0.001000
  EtherCAT PDO Receive16 : xpcethercatlib/EtherCAT PDO Receive  Priority=2  sig_name=Box 6 (ATRIAS 2.1 Leg (Medulla 1.5)).Thermistors.Thermistor 4  sig_offset=1872  sig_type=uint16  type_size=16  sig_dim=1  device_id=0  sample_time=0.001000
  EtherCAT PDO Receive17 : xpcethercatlib/EtherCAT PDO Receive  Priority=2  sig_name=Box 6 (ATRIAS 2.1 Leg (Medulla 1.5)).Thermistors.Thermistor 5  sig_offset=1888  sig_type=uint16  type_size=16  sig_dim=1  device_id=0  sample_time=0.001000
  EtherCAT PDO Receive18 : xpcethercatlib/EtherCAT PDO Receive  Priority=2  sig_name=Box 6 (ATRIAS 2.1 Leg (Medulla 1.5)).uController Status.Counter  sig_offset=1608  sig_type=uint8  type_size=8  sig_dim=1  device_id=0  sample_time=0.001000
  EtherCAT PDO Receive19 : xpcethercatlib/EtherCAT PDO Receive  Priority=2  sig_name=Box 6 (ATRIAS 2.1 Leg (Medulla 1.5)).uController Status.Error Flags  sig_offset=1616  sig_type=uint8  type_size=8  sig_dim=1  device_id=0  sample_time=0.001000
  EtherCAT PDO Receive2 : xpcethercatlib/EtherCAT PDO Receive  Priority=2  sig_name=Box 6 (ATRIAS 2.1 Leg (Medulla 1.5)).Knee Force.Knee Force 1  sig_offset=1936  sig_type=uint16  type_size=16  sig_dim=1  device_id=0  sample_time=0.001000
  EtherCAT PDO Receive20 : xpcethercatlib/EtherCAT PDO Receive  Priority=2  sig_name=Box 6 (ATRIAS 2.1 Leg (Medulla 1.5)).uController Status.ID  sig_offset=1592  sig_type=uint8  type_size=8  sig_dim=1  device_id=0  sample_time=0.001000
  EtherCAT PDO Receive21 : xpcethercatlib/EtherCAT PDO Receive  Priority=2  sig_name=Box 6 (ATRIAS 2.1 Leg (Medulla 1.5)).uController Status.State  sig_offset=1600  sig_type=uint8  type_size=8  sig_dim=1  device_id=0  sample_time=0.001000
  EtherCAT PDO Receive22 : xpcethercatlib/EtherCAT PDO Receive  Priority=2  sig_name=Box 6 (ATRIAS 2.1 Leg (Medulla 1.5)).uController Status.Limit Switch  sig_offset=1624  sig_type=uint8  type_size=8  sig_dim=1  device_id=0  sample_time=0.001000
  EtherCAT PDO Receive23 : xpcethercatlib/EtherCAT PDO Receive  Priority=2  sig_name=Box 6 (ATRIAS 2.1 Leg (Medulla 1.5)).uController Status.Toe Sensor  sig_offset=1632  sig_type=uint16  type_size=16  sig_dim=1  device_id=0  sample_time=0.001000
  EtherCAT PDO Receive3 : xpcethercatlib/EtherCAT PDO Receive  Priority=2  sig_name=Box 6 (ATRIAS 2.1 Leg (Medulla 1.5)).Knee Force.Knee Force 2  sig_offset=1952  sig_type=uint16  type_size=16  sig_dim=1  device_id=0  sample_time=0.001000
  EtherCAT PDO Receive4 : xpcethercatlib/EtherCAT PDO Receive  Priority=2  sig_name=Box 6 (ATRIAS 2.1 Leg (Medulla 1.5)).Leg Encoder.Leg Encoder  sig_offset=1696  sig_type=uint32  type_size=32  sig_dim=1  device_id=0  sample_time=0.001000
  EtherCAT PDO Receive5 : xpcethercatlib/EtherCAT PDO Receive  Priority=2  sig_name=Box 6 (ATRIAS 2.1 Leg (Medulla 1.5)).Leg Encoder.Leg Encoder Timestamp  sig_offset=1728  sig_type=uint16  type_size=16  sig_dim=1  device_id=0  sample_time=0.001000
  EtherCAT PDO Receive6 : xpcethercatlib/EtherCAT PDO Receive  Priority=2  sig_name=Box 6 (ATRIAS 2.1 Leg (Medulla 1.5)).Measured Current.Amp 1 Measured Current  sig_offset=1904  sig_type=int16  type_size=16  sig_dim=1  device_id=0  sample_time=0.001000
  EtherCAT PDO Receive7 : xpcethercatlib/EtherCAT PDO Receive  Priority=2  sig_name=Box 6 (ATRIAS 2.1 Leg (Medulla 1.5)).Measured Current.Amp 2 Measured Current  sig_offset=1920  sig_type=int16  type_size=16  sig_dim=1  device_id=0  sample_time=0.001000
  EtherCAT PDO Receive8 : xpcethercatlib/EtherCAT PDO Receive  Priority=2  sig_name=Box 6 (ATRIAS 2.1 Leg (Medulla 1.5)).Motor Encoder.Motor Encoder  sig_offset=1648  sig_type=uint32  type_size=32  sig_dim=1  device_id=0  sample_time=0.001000
  EtherCAT PDO Receive9 : xpcethercatlib/EtherCAT PDO Receive  Priority=2  sig_name=Box 6 (ATRIAS 2.1 Leg (Medulla 1.5)).Motor Encoder.Motor Encoder Timestamp  sig_offset=1680  sig_type=uint16  type_size=16  sig_dim=1  device_id=0  sample_time=0.001000
  EtherCAT PDO Transmit : xpcethercatlib/EtherCAT PDO Transmit   Priority=3  sig_name=Box 6 (ATRIAS 2.1 Leg (Medulla 1.5)).uControllerInput.Command  sig_offset=1592  sig_type=uint8  type_size=8  sig_dim=1  device_id=0  sample_time=0.001000
  EtherCAT PDO Transmit1 : xpcethercatlib/EtherCAT PDO Transmit   Priority=3  sig_name=Box 6 (ATRIAS 2.1 Leg (Medulla 1.5)).uControllerInput.Counter  sig_offset=1600  sig_type=uint16  type_size=16  sig_dim=1  device_id=0  sample_time=0.001000
  EtherCAT PDO Transmit2 : xpcethercatlib/EtherCAT PDO Transmit   Priority=3  Commented=on  sig_name=Box 6 (ATRIAS 2.1 Leg (Medulla 1.5)).uControllerInput.Motor Current  sig_offset=1616  sig_type=int32  type_size=32  sig_dim=1  device_id=0  sample_time=0.001000
  EtherCAT PDO Transmit3 : xpcethercatlib/EtherCAT PDO Transmit   Priority=3  sig_name=Box 6 (ATRIAS 2.1 Leg (Medulla 1.5)).uControllerInput.Motor Current  sig_offset=1616  sig_type=int32  type_size=32  sig_dim=1  device_id=0  sample_time=0.001000
  Gain : Gain  Commented=on  Gain=1e9
  "Session Time " : slrtlib/Target Management/Target Information/Session Time   Commented=on  ts=0.001
  LegEncoder : Outport
  MotorEncoder : Outport  Port=2
  ToeSensor : Outport  Port=3
  LimitSwitch : Outport  Port=4
  ID : Outport  Port=5
  State : Outport  Port=6
  Counter : Outport  Port=7
  ErrorFlags : Outport  Port=8
  IncEncoder : Outport  Port=9
  LegEncoderTimestamp : Outport  Port=10
  MotorEncoderTimestamp : Outport  Port=11
  IncEncoderTimestamp : Outport  Port=12
  MotorVoltage : Outport  Port=13
  LogicVoltage : Outport  Port=14
  Thermistor0 : Outport  Port=15
  Thermistor1 : Outport  Port=16
  Thermistor2 : Outport  Port=17
  Thermistor3 : Outport  Port=18
  Thermistor4 : Outport  Port=19
  Thermistor5 : Outport  Port=20
  Amp1MeasuredCurrent : Outport  Port=21
  Amp2MeasuredCurrent : Outport  Port=22
  KneeForce1 : Outport  Port=23
  KneeForce2 : Outport  Port=24
  counter send : Outport  Port=25
  execution time : Outport  Port=26
  wires:
  Data Type Conversion/1 -> EtherCAT PDO Transmit/1
  Data Type Conversion1/1 -> EtherCAT PDO Transmit1/1
  Data Type Conversion2/1 -> ?
  EtherCAT PDO Receive/1 -> IncEncoder/1
  EtherCAT PDO Receive1/1 -> IncEncoderTimestamp/1
  EtherCAT PDO Receive2/1 -> KneeForce1/1
  EtherCAT PDO Receive3/1 -> KneeForce2/1
  EtherCAT PDO Receive4/1 -> LegEncoder/1
  EtherCAT PDO Receive5/1 -> LegEncoderTimestamp/1
  EtherCAT PDO Receive6/1 -> Amp1MeasuredCurrent/1
  EtherCAT PDO Receive7/1 -> Amp2MeasuredCurrent/1
  EtherCAT PDO Receive8/1 -> MotorEncoder/1
  EtherCAT PDO Receive9/1 -> MotorEncoderTimestamp/1
  EtherCAT PDO Receive10/1 -> LogicVoltage/1
  EtherCAT PDO Receive11/1 -> MotorVoltage/1
  EtherCAT PDO Receive12/1 -> Thermistor0/1
  EtherCAT PDO Receive13/1 -> Thermistor1/1
  EtherCAT PDO Receive14/1 -> Thermistor2/1
  EtherCAT PDO Receive15/1 -> Thermistor3/1
  EtherCAT PDO Receive16/1 -> Thermistor4/1
  EtherCAT PDO Receive17/1 -> Thermistor5/1
  EtherCAT PDO Receive18/1 -> Counter/1
  EtherCAT PDO Receive19/1 -> ErrorFlags/1
  EtherCAT PDO Receive20/1 -> ID/1
  EtherCAT PDO Receive22/1 -> LimitSwitch/1
  EtherCAT PDO Receive21/1 -> State/1
  EtherCAT PDO Receive23/1 -> ToeSensor/1
  MedullaCmd/1 -> Data Type Conversion/1
  MedullaCounter/1 -> Data Type Conversion1/1
  MotorCmd/1 -> Data Type Conversion2/1
  Data Type Conversion3/1 -> EtherCAT PDO Transmit2/1, counter send/1
  Gain/1 -> Data Type Conversion3/1, execution time/1
  "Session Time "/1 -> Gain/1

== system atrias_system_testing_delay/DAQ/calibrate_and_convert_to_rad ==
  encoder_ticks : Inport
  Constant : Constant  Value=-HIP_INC_ENCODER_RAD_PER_TICK
  Constant1 : Constant  Value=HIP_INC_ENCODER_RAD_PER_TICK
  Constant2 : Constant  Value=BOOM_YAW_ENCODER_RAD_PER_TICK
  Mux1 : Mux  Inputs=2
  Mux2 : Mux  Inputs=3
  Product : Product  RndMeth=Zero
  Selector1 : Selector  InputPortWidth=3  Indices=[1 2]
  Selector2 : Selector  InputPortWidth=15  Indices=[1 2 3 4 5 6 7 8 9 10 11 15 12]
  calibrate_abs_encoder : Subsystem
  calibration_pt_radians : Subsystem
  calibration_pt_ticks : Subsystem
  select_abs : Selector  InputPortWidth=15  Indices=[1 2 3 4 5 6 7 8 9 11 13 15]
  select_inc : Selector  InputPortWidth=15  Indices=[10 12 14]
  ticks_to_radians_constants : Subsystem
  q : Outport
  hip_inc : Outport  Port=2
  wires:
  Constant2/1 -> Mux2/3
  Constant1/1 -> Mux2/2
  Constant/1 -> Mux2/1
  Product/1 -> Mux1/2, Selector1/1
  Mux2/1 -> Product/2
  select_inc/1 -> Product/1
  Selector2/1 -> q/1
  Mux1/1 -> Selector2/1
  select_abs/1 -> calibrate_abs_encoder/1(encoder_ticks)
  calibrate_abs_encoder/1(angle [rad]) -> Mux1/1
  ticks_to_radians_constants/1(ticks_to_rad_constants) -> calibrate_abs_encoder/4(ticks_to_rad_const)
  calibration_pt_radians/1(calibration_pt [rad]) -> calibrate_abs_encoder/3(cal_pt_rad)
  calibration_pt_ticks/1(calibration_pt [ticks]) -> calibrate_abs_encoder/2(cal_pt_ticks)
  encoder_ticks/1 -> select_abs/1, select_inc/1
  Selector1/1 -> hip_inc/1

== system atrias_system_testing_delay/DAQ/low_pass_derivative ==
  q : Inport
  hip_inc : Inport  Port=2
  timestamps : Inport  Port=3
  Add : Sum
  Constant : Constant  Value=nom_sample_time
  Constant1 : Constant  Value=MEDULLA_TIMER_FREQ
  Divide : Product  Inputs=*/
  Divide1 : Product  Inputs=*/
  Mux : Mux  Inputs=2
  Selector2 : Selector  InputPortWidth=15  Indices=[1:8 14:15 11:13]
  difference : simulink/Discrete/Difference  ICPrevInput=0.0  InputProcessing=Inherited  OutMin=[]  OutMax=[]  OutDataType=fixdt(1, 16)  OutScaling=2^-10  DoSatur=off
  difference1 : simulink/Discrete/Difference  ICPrevInput=0.0  InputProcessing=Inherited  OutMin=[]  OutMax=[]  OutDataType=fixdt(1, 16)  OutScaling=2^-10  DoSatur=off
  two_pole_filter : DiscreteTransferFcn  Numerator=[A_lpf_velocity 0 0]  Denominator=[1 B1_lpf_velocity B2_lpf_velocity]  SampleTime=sample_time
  dq : Outport
  wires:
  q/1 -> Mux/1
  hip_inc/1 -> Mux/2
  Mux/1 -> Selector2/1
  Selector2/1 -> difference/1
  difference/1 -> Divide/1
  timestamps/1 -> difference1/1
  difference1/1 -> Divide1/1
  Constant1/1 -> Divide1/2
  Constant/1 -> Add/1
  Divide1/1 -> Add/2
  Add/1 -> Divide/2
  Divide/1 -> dq/1

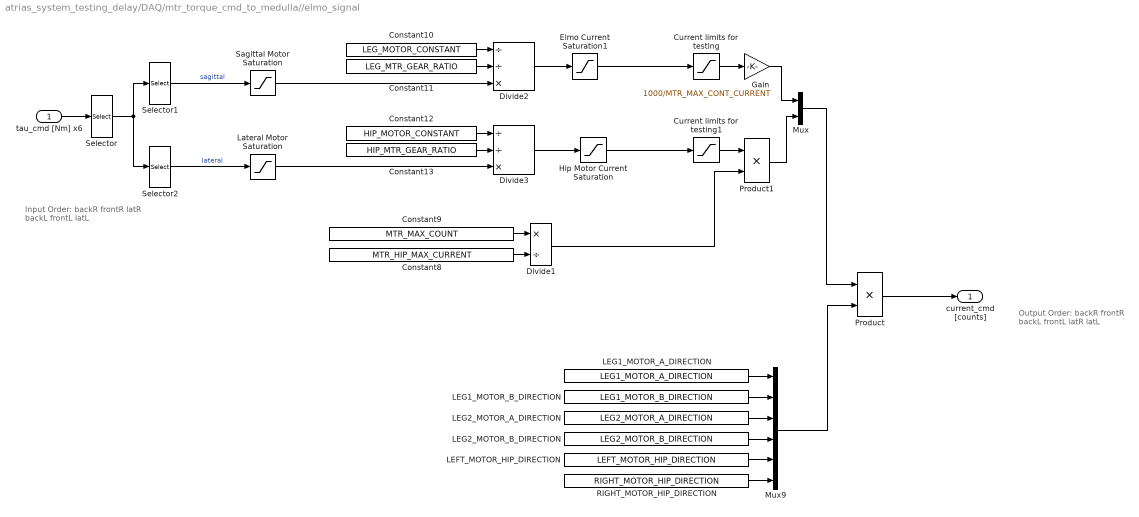
== system atrias_system_testing_delay/DAQ/mtr_torque_cmd_to_medulla//elmo_signal ==
  note: Output Order:
      |
      | backR
      | frontR
      | backL
      | frontL
      | latR
      | latL
  note: Input Order:
      |
      | backR
      | frontR
      | latR
      | backL
      | frontL
      | latL
  tau_cmd [Nm] x6 : Inport
  Constant10 : Constant  Value=LEG_MOTOR_CONSTANT
  Constant11 : Constant  Value=LEG_MTR_GEAR_RATIO
  Constant12 : Constant  Value=HIP_MOTOR_CONSTANT
  Constant13 : Constant  Value=HIP_MTR_GEAR_RATIO
  Constant8 : Constant  Value=MTR_HIP_MAX_CURRENT
  Constant9 : Constant  Value=MTR_MAX_COUNT
  Current limits for testing : Saturate  UpperLimit=CURRENT_LIMIT  LowerLimit=-CURRENT_LIMIT
      settings: AttributesFormatString=Top: %<UpperLimit>\nBottom: %<LowerLimit>
  Current limits for testing1 : Saturate  UpperLimit=CURRENT_LIMIT  LowerLimit=-CURRENT_LIMIT
      settings: AttributesFormatString=Top: %<UpperLimit>\nBottom: %<LowerLimit>
  Divide1 : Product  Inputs=*/
  Divide2 : Product  Inputs=//*
  Divide3 : Product  Inputs=//*
  Elmo Current Saturation1 : Saturate  UpperLimit=MTR_MAX_CURRENT  LowerLimit=-MTR_MAX_CURRENT
      settings: AttributesFormatString=Top: %<UpperLimit>\nBottom: %<LowerLimit>
  Gain : Gain  Gain=1000/MTR_MAX_CONT_CURRENT
  Hip Motor Current Saturation : Saturate  UpperLimit=MTR_HIP_MAX_CURRENT  LowerLimit=-MTR_HIP_MAX_CURRENT
      settings: AttributesFormatString=Top: %<UpperLimit>\nBottom: %<LowerLimit>
  LEFT_MOTOR_HIP_DIRECTION : Constant  Value=LEFT_MOTOR_HIP_DIRECTION
  LEG1_MOTOR_A_DIRECTION : Constant  Value=LEG1_MOTOR_A_DIRECTION
  LEG1_MOTOR_B_DIRECTION : Constant  Value=LEG1_MOTOR_B_DIRECTION
  LEG2_MOTOR_A_DIRECTION : Constant  Value=LEG2_MOTOR_A_DIRECTION
  LEG2_MOTOR_B_DIRECTION : Constant  Value=LEG2_MOTOR_B_DIRECTION
  Lateral Motor Saturation : Saturate  UpperLimit=HIP_MTR_MAX_TORQUE  LowerLimit=-HIP_MTR_MAX_TORQUE
      settings: AttributesFormatString=Top: %<UpperLimit>\nBottom: %<LowerLimit>
  Mux : Mux  Inputs=2
  Mux9 : Mux  Inputs=6
  Product : Product  RndMeth=Zero
  Product1 : Product  RndMeth=Zero
  RIGHT_MOTOR_HIP_DIRECTION : Constant  Value=RIGHT_MOTOR_HIP_DIRECTION
  Sagittal Motor Saturation : Saturate  UpperLimit=LEG_MTR_MAX_TORQUE  LowerLimit=-LEG_MTR_MAX_TORQUE
      settings: AttributesFormatString=Top: %<UpperLimit>\nBottom: %<LowerLimit>
  Selector : Selector  InputPortWidth=6  Indices=[1 2 4 5 3 6]
  Selector1 : Selector  InputPortWidth=6  Indices=[1 2 3 4]
  Selector2 : Selector  InputPortWidth=6  Indices=[5 6]
  current_cmd [counts] : Outport
  wires:
  Lateral Motor Saturation/1 -> Divide3/3
  Sagittal Motor Saturation/1 -> Divide2/3
  Gain/1 -> Mux/1
  Mux/1 -> Product/1
  Divide2/1 -> Elmo Current Saturation1/1
  Constant12/1 -> Divide3/1
  Constant13/1 -> Divide3/2
  Constant10/1 -> Divide2/1
  Constant11/1 -> Divide2/2
  Selector2/1 -> Lateral Motor Saturation/1  "lateral"
  Selector1/1 -> Sagittal Motor Saturation/1  "sagittal"
  LEG1_MOTOR_A_DIRECTION/1 -> Mux9/1
  LEG1_MOTOR_B_DIRECTION/1 -> Mux9/2
  LEG2_MOTOR_A_DIRECTION/1 -> Mux9/3
  Mux9/1 -> Product/2
  LEG2_MOTOR_B_DIRECTION/1 -> Mux9/4
  LEFT_MOTOR_HIP_DIRECTION/1 -> Mux9/5
  RIGHT_MOTOR_HIP_DIRECTION/1 -> Mux9/6
  Product/1 -> current_cmd [counts]/1
  tau_cmd [Nm] x6/1 -> Selector/1
  Selector/1 -> Selector1/1, Selector2/1
  Hip Motor Current Saturation/1 -> Current limits for testing1/1
  Divide3/1 -> Hip Motor Current Saturation/1
  Constant9/1 -> Divide1/1
  Constant8/1 -> Divide1/2
  Divide1/1 -> Product1/2
  Elmo Current Saturation1/1 -> Current limits for testing/1
  Product1/1 -> Mux/2
  Current limits for testing1/1 -> Product1/1
  Current limits for testing/1 -> Gain/1

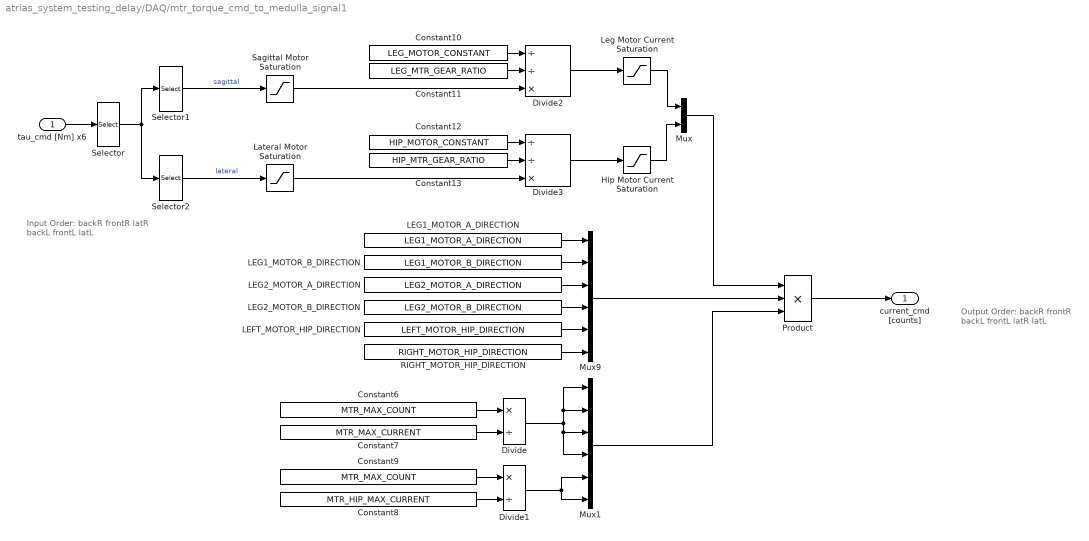
== system atrias_system_testing_delay/DAQ/mtr_torque_cmd_to_medulla_signal1 ==
  note: Output Order:
      |
      | backR
      | frontR
      | backL
      | frontL
      | latR
      | latL
  note: Input Order:
      |
      | backR
      | frontR
      | latR
      | backL
      | frontL
      | latL
  tau_cmd [Nm] x6 : Inport
  Constant10 : Constant  Value=LEG_MOTOR_CONSTANT
  Constant11 : Constant  Value=LEG_MTR_GEAR_RATIO
  Constant12 : Constant  Value=HIP_MOTOR_CONSTANT
  Constant13 : Constant  Value=HIP_MTR_GEAR_RATIO
  Constant6 : Constant  Value=MTR_MAX_COUNT
  Constant7 : Constant  Value=MTR_MAX_CURRENT
  Constant8 : Constant  Value=MTR_HIP_MAX_CURRENT
  Constant9 : Constant  Value=MTR_MAX_COUNT
  Divide : Product  Inputs=*/
  Divide1 : Product  Inputs=*/
  Divide2 : Product  Inputs=//*
  Divide3 : Product  Inputs=//*
  Hip Motor Current Saturation : Saturate  UpperLimit=10  LowerLimit=-10
      settings: AttributesFormatString=Top: %<UpperLimit>\nBottom: %<LowerLimit>
  LEFT_MOTOR_HIP_DIRECTION : Constant  Value=LEFT_MOTOR_HIP_DIRECTION
  LEG1_MOTOR_A_DIRECTION : Constant  Value=LEG1_MOTOR_A_DIRECTION
  LEG1_MOTOR_B_DIRECTION : Constant  Value=LEG1_MOTOR_B_DIRECTION
  LEG2_MOTOR_A_DIRECTION : Constant  Value=LEG2_MOTOR_A_DIRECTION
  LEG2_MOTOR_B_DIRECTION : Constant  Value=LEG2_MOTOR_B_DIRECTION
  Lateral Motor Saturation : Saturate  UpperLimit=HIP_MTR_MAX_TORQUE  LowerLimit=-HIP_MTR_MAX_TORQUE
      settings: AttributesFormatString=Top: %<UpperLimit>\nBottom: %<LowerLimit>
  Leg Motor Current Saturation : Saturate  UpperLimit=60  LowerLimit=-60
      settings: AttributesFormatString=Top: %<UpperLimit>\nBottom: %<LowerLimit>
  Mux : Mux  Inputs=2
  Mux1 : Mux  Inputs=6
  Mux9 : Mux  Inputs=6
  Product : Product  Inputs=3  RndMeth=Zero
  RIGHT_MOTOR_HIP_DIRECTION : Constant  Value=RIGHT_MOTOR_HIP_DIRECTION
  Sagittal Motor Saturation : Saturate  UpperLimit=LEG_MTR_MAX_TORQUE  LowerLimit=-LEG_MTR_MAX_TORQUE
      settings: AttributesFormatString=Top: %<UpperLimit>\nBottom: %<LowerLimit>
  Selector : Selector  InputPortWidth=6  Indices=[1 2 4 5 3 6]
  Selector1 : Selector  InputPortWidth=6  Indices=[1 2 3 4]
  Selector2 : Selector  InputPortWidth=6  Indices=[5 6]
  current_cmd [counts] : Outport
  wires:
  Lateral Motor Saturation/1 -> Divide3/3
  Sagittal Motor Saturation/1 -> Divide2/3
  Hip Motor Current Saturation/1 -> Mux/2
  Leg Motor Current Saturation/1 -> Mux/1
  Mux/1 -> Product/1
  Divide2/1 -> Leg Motor Current Saturation/1
  Divide3/1 -> Hip Motor Current Saturation/1
  Constant12/1 -> Divide3/1
  Constant13/1 -> Divide3/2
  Constant10/1 -> Divide2/1
  Constant11/1 -> Divide2/2
  Selector2/1 -> Lateral Motor Saturation/1  "lateral"
  Selector1/1 -> Sagittal Motor Saturation/1  "sagittal"
  LEG1_MOTOR_A_DIRECTION/1 -> Mux9/1
  LEG1_MOTOR_B_DIRECTION/1 -> Mux9/2
  LEG2_MOTOR_A_DIRECTION/1 -> Mux9/3
  Mux9/1 -> Product/2
  LEG2_MOTOR_B_DIRECTION/1 -> Mux9/4
  LEFT_MOTOR_HIP_DIRECTION/1 -> Mux9/5
  RIGHT_MOTOR_HIP_DIRECTION/1 -> Mux9/6
  Product/1 -> current_cmd [counts]/1
  Constant6/1 -> Divide/1
  Constant7/1 -> Divide/2
  Divide/1 -> Mux1/4, Mux1/3, Mux1/2, Mux1/1
  Constant9/1 -> Divide1/1
  Constant8/1 -> Divide1/2
  Divide1/1 -> Mux1/6, Mux1/5
  Mux1/1 -> Product/3
  tau_cmd [Nm] x6/1 -> Selector/1
  Selector/1 -> Selector1/1, Selector2/1

== system atrias_system_testing_delay/DAQ/remove_encoder_dropouts ==
  note: predicted value:
      | phi' = phi_(n-1) + dphi
      | = phi_(n-1) + phi_(n-1)-phi_(n-2)
  note: Predict Behavior of Signal
  measured : Inport
  Abs : Abs
  Clock : Clock
  Compare To Zero1 : simulink/Logic and Bit Operations/Compare To Zero  relop=>  OutDataTypeStr=boolean
  Constant : Constant  Value=sensor_start_time+2*sample_time
  Discrete Single Pole Lowpass Filter : DiscreteTransferFcn  Numerator=[(1-exp(-2*pi*fcut_smooth*sample_time)) 0]  Denominator=[1 -exp(-2*pi*fcut_smooth*sample_time)]  SampleTime=sample_time
  Gain2 : Gain  Gain=2
  Sum : Sum  Inputs=|+-
  Sum2 : Sum  Inputs=|+-
  Sum3 : Sum  Inputs=-+|
  Switch : Switch  Criteria=u2 ~= 0  Threshold=max_sensor_velocity*sample_time
      settings: AttributesFormatString=%<Criteria>
  Unit Delay phi_(n-1) : UnitDelay  SampleTime=-1
      settings: AttributesFormatString=initial condition = %<X0>
  Unit Delay phi_(n-2) : UnitDelay  SampleTime=-1
      settings: AttributesFormatString=initial condition = %<X0>
  check_error : Subsystem
  smoothed : Outport
  wires:
  Sum/1 -> Switch/3, Sum3/2  "phi'"
  Gain2/1 -> Sum/1
  Unit Delay phi_(n-1)/1 -> Gain2/1, Unit Delay phi_(n-2)/1
  measured/1 -> Sum3/1, Switch/1  "phi"
  Unit Delay phi_(n-2)/1 -> Sum/2
  Switch/1 -> Discrete Single Pole Lowpass Filter/1, smoothed/1
  Discrete Single Pole Lowpass Filter/1 -> Unit Delay phi_(n-1)/1
  Abs/1 -> check_error/1(error)
  Sum3/1 -> Abs/1  "error"
  check_error/1(acceptable?) -> Switch/2
  Sum2/1 -> Compare To Zero1/1
  Clock/1 -> Sum2/1
  Constant/1 -> Sum2/2
  Compare To Zero1/1 -> check_error/Enable

== system atrias_system_testing_delay/DAQ/unwrap_encoders ==
  Encoder Readings : Inport
  Demux : Demux  Outputs=5
  Mux : Mux  Inputs=6
  Selector : Selector  InputPortWidth=15  Indices=[9 10 11 12 14]
  Selector1 : Selector  InputPortWidth=20  Indices=[1 2 3 4 5 6 7 8 16 17 18 19 13 20 15]
  unwrap_boom_yaw_encoder : Subsystem
  unwrap_lateral_absolute_encoders Left : Subsystem
  unwrap_lateral_absolute_encoders Right : Subsystem
  unwrap_lateral_incremental_encoders Left : Subsystem
  unwrap_lateral_incremental_encoders Right : Subsystem
  Adjusted Encoder Readings : Outport
  wires:
  unwrap_lateral_absolute_encoders Left/1(continuous [ticks]) -> Mux/4
  Demux/3 -> unwrap_lateral_absolute_encoders Left/1(wrapped [ticks])
  Demux/1 -> unwrap_lateral_absolute_encoders Right/1(wrapped [ticks])
  Mux/1 -> Selector1/1
  Selector1/1 -> Adjusted Encoder Readings/1
  unwrap_boom_yaw_encoder/1(continuous [ticks]) -> Mux/6
  unwrap_lateral_incremental_encoders Left/1(continuous [ticks]) -> Mux/5
  unwrap_lateral_incremental_encoders Right/1(continuous [ticks]) -> Mux/3
  Demux/5 -> unwrap_boom_yaw_encoder/1(wrapped [ticks])
  Demux/4 -> unwrap_lateral_incremental_encoders Left/1(wrapped [ticks])
  Demux/2 -> unwrap_lateral_incremental_encoders Right/1(wrapped [ticks])
  Selector/1 -> Demux/1
  Encoder Readings/1 -> Selector/1, Mux/1
  unwrap_lateral_absolute_encoders Right/1(continuous [ticks]) -> Mux/2

== system atrias_system_testing_delay/Start Controller/Hold Start Time ==
  Time In : Inport  OutDataTypeStr=double
  Enable : EnablePort
  Time Out : Outport  OutDataTypeStr=double
  wires:
  Time In/1 -> Time Out/1

== system atrias_system_testing_delay/DAQ/Elmo Back Left/Drive state transition ==
  Status : Inport
  Bitwise Operator : simulink/Logic and Bit Operations/Bitwise Operator  logicop=AND  UseBitMask=on  BitMask=hex2dec('ff')  BitMaskRealWorld=Stored Integer
  Bitwise Operator1 : simulink/Logic and Bit Operations/Bitwise Operator  logicop=AND  UseBitMask=on  BitMask=hex2dec('80')  BitMaskRealWorld=Stored Integer
  Compare To Constant : simulink/Logic and Bit Operations/Compare To Constant  relop===  const=80  OutDataTypeStr=boolean
  Compare To Constant1 : simulink/Logic and Bit Operations/Compare To Constant  relop===  const=49  OutDataTypeStr=boolean
  Compare To Constant2 : simulink/Logic and Bit Operations/Compare To Constant  relop===  const=51  OutDataTypeStr=boolean
  Compare To Constant3 : simulink/Logic and Bit Operations/Compare To Constant  relop===  const=55  OutDataTypeStr=boolean
  Compare To Zero : simulink/Logic and Bit Operations/Compare To Zero  relop=~=  OutDataTypeStr=boolean
  Constant : Constant  Value=0  OutDataTypeStr=uint16
  Constant1 : Constant  Value=128  OutDataTypeStr=uint16
  Constant2 : Constant  Value=6  OutDataTypeStr=uint16
  Constant3 : Constant  Value=7  OutDataTypeStr=uint16
  Constant4 : Constant  Value=15  OutDataTypeStr=uint16
  Constant5 : Constant  Value=15  OutDataTypeStr=uint16
  Switch{,1..4} (5 alike) : Switch  Criteria=u2 > Threshold
  Control : Outport
  wires:
  Status/1 -> Bitwise Operator/1, Bitwise Operator1/1
  Bitwise Operator1/1 -> Compare To Zero/1
  Compare To Zero/1 -> Switch/2
  Constant1/1 -> Switch/1
  Constant/1 -> Switch/3
  Compare To Constant/1 -> Switch1/2
  Switch/1 -> Switch1/3
  Bitwise Operator/1 -> Compare To Constant3/1, Compare To Constant2/1, Compare To Constant1/1, Compare To Constant/1
  Constant2/1 -> Switch1/1
  Compare To Constant1/1 -> Switch2/2
  Switch1/1 -> Switch2/3
  Constant3/1 -> Switch2/1
  Compare To Constant2/1 -> Switch3/2
  Switch2/1 -> Switch3/3
  Constant4/1 -> Switch3/1
  Compare To Constant3/1 -> Switch4/2
  Switch3/1 -> Switch4/3
  Constant5/1 -> Switch4/1
  Switch4/1 -> Control/1
